simulink model "Bands6"  (R2018a)
settings: Solver=VariableStepAuto  StartTime=0.0  StopTime=0.01  RelTol=1e-3
undefined symbols (not defined in the file): fdesignblkfcn, G1, G2, G3, G4, G5, G6, gcbh, get, T
libraries: dspsrcs4 x1, dspxfrm3 x1, dspobslib x1
(part 2 of 2)

== system Bands6/Filter Bank /Filter 5/Bandpass Filter ==
  In : Inport
  Generated Filter Block : DiscreteFir  Tag=BlockMethodSubSystem  Coefficients=[5.80169645545239008e-08 -7.36943237726898499e-08 -1.75427224261787647e-07 6.43003652238008357e-07 -5.28400861014822699e-07 -1.09677006372124872e-06 3.31781145815797723e-06 -2.53629827715104648e-06 -3.9844890702122352e-06 1.18719656898654724e-05 -9.36329870334377579e-06 -1.03790001202894647e-05 3.33782074792234292e-05 -2.82688496798137121e-05 -2.05521184487442067e-05 7.80506937687390717e-05 -7.24051531518292809e-05 -3.00972665896463103e-05 0.000156331642592978074 -0.000161139708449589659 -2.51459625490565774e-05 0.00027208320875304079 -0.000316608173078618781 2.16589686587504518e-05 0.000412616192629136256 -0.000554862993402606202 0.000150692654732448582 0.000539329012231355752 -0.000872369046581383074 0.00040648652621871461 0.000585591917311480354 -0.00123249299141194816 0.000819163333665229158 0.000468918632894233629 -0.00156026749336166831 0.00138023742307578651 0.000120378783589651138 -0.00175423169147518113 0.0020230393593841569 -0.000474494460511202902 -0.00171910430407683527 0.00262123067921987652 -0.00123929489922535211 -0.00141248066958475638 0.00301527620477055891 -0.00199678966571106148 -0.000886619376992856694 0.00306523259567484602 -0.00250307330187033404 -0.000299861672526029936 0.00271252560159371226 -0.0025267776534030565 0.00012171384745463444 0.00202172673597837823 -0.00195008342165233677 0.000171258457679733067 0.00117467533990653263 -0.000848223237854478789 -0.000232692021354291518 0.000407587462984154323 0.00049828682517694795 -0.000971874699162834465 -8.85610034070924331e-05 0.00168202383752096766 -0.00173587675048004716 -0.000257954610305697056 0.00231927882960823771 -0.0021311939810607387 -0.000208481271414066242 0.00221255995829579624 -0.00186005918159203617 -0.000152015535511321729 0.00144662698791519725 -0.000889902743837175589 -0.000276867996253072691 0.000361608279357888897 0.000479878382522087887 -0.000618501588275072352 -0.000596003608316242437 0.00171105795524934576 -0.00100922150237675286 -0.00107795666262090685 0.00225971295712451125 -0.00115432392189464793 -0.000990924709133747398 0.00184772697412779606 -0.000811329556474037271 -0.000519796048615203871 0.000632035063372947707 2.24795851541013272e-05 -1.99606835156976085e-06 -0.000834109638794323189 0.00103494686315405552 0.000276818419330519436 -0.00185226591461002538 0.0017108115780006762 0.000244592720617982785 -0.00192809879322400628 0.00160075014399831887 6.14690263060736021e-05 -0.00103627337936797875 0.000611243434872120656 -1.91465685851059381e-05 0.000352130594981162352 -0.00086254312190905296 0.000142472563550124576 0.00151075077237486713 -0.00207507689699802569 0.000441166590936414166 0.00184666137896536179 -0.00230619796031119239 0.000576883090156487025 0.0012222015245354689 -0.00128685755170820796 0.000274230407592072759 2.27936196504474287e-05 0.000575424432464703099 -0.000466214697355777784 -0.0010743474392980398 0.00233874424726945645 -0.00127094741825165588 -0.00149764925353861132 0.00300421201905462943 -0.00156043086177853007 -0.00110627437447876828 0.00208716316600946047 -0.000919833301459701278 -0.000243179188607324851 -4.7857526112472211e-05 0.000546643345120831196 0.00051568179032762348 -0.00231508901657014434 0.00213514192708850938 0.000751567312124432063 -0.0034701576132279803 0.00285729371205205957 0.000471220012500609764 -0.00281293450406624882 0.00202632646388123307 6.63362851220782198e-05 -0.000623898569242482153 -0.000221229277446687944 -1.44191510628433379e-05 0.00194568773553285574 -0.00282840865428083277 0.00034940405710216229 0.00349933860496167174 -0.00429430022970904175 0.000800524320988185841 0.00319057761487220827 -0.00352540131711092655 0.000738596481679123563 0.00121803959086664378 -0.000585118425519459435 -0.000185229365218113291 -0.0012888920303765674 0.00315005677366268387 -0.00165923705179339448 -0.00294013727937736304 0.00562004228208647615 -0.00273360598608378934 -0.00290891244731987606 0.00522195115943085032 -0.00236421374140658282 -0.00139899652620957245 0.00182892903336386633 ...(+7522 chars)]  InputProcessing=Columns as channels (frame based)
  Out : Outport
  wires:
  In/1 -> Generated Filter Block/1
  Generated Filter Block/1 -> Out/1

== system Bands6/Filter Bank /Filter 6/Bandpass Filter ==
  In : Inport
  Generated Filter Block : DiscreteFir  Tag=BlockMethodSubSystem  Coefficients=[-8.46163060201177932e-08 4.43935124807243188e-07 -1.41960685880143677e-06 3.41720796909821398e-06 -6.66356512995420131e-06 1.08407356256788048e-05 -1.47502152166903733e-05 1.62989488752967176e-05 -1.30606215944798934e-05 3.47793268459825403e-06 1.16523753158832859e-05 -2.8158246186184923e-05 3.88640762038403156e-05 -3.59073795891534178e-05 1.46745586998780423e-05 2.21494551041817479e-05 -6.26963714884166994e-05 8.82752874711505939e-05 -8.04749647169068934e-05 3.10014021065765821e-05 5.01508359255908656e-05 -0.000133325946508563016 0.000177869540798289167 -0.000149597937610631751 4.05769804763433638e-05 0.000118706402074483244 -0.000263643793305792513 0.000318902583301029741 -0.000233976101207557848 1.54785793754956013e-05 0.000261673317368628204 -0.000475446213967466928 0.000507183945928171539 -0.000302117535111148827 -8.9147778119413865e-05 0.000513780824357670698 -0.000772340819809743035 0.00070904989012480742 -0.000297360294473450167 -0.000323673059816665851 0.000889607105286156145 -0.00112031835339431742 0.00085533138476342216 -0.000150635139510927289 -0.000717538205679782003 0.00135740149880777552 -0.00143743203462967997 0.000854983806421841328 0.00018714488152558458 -0.00124511234139790998 0.00182327158032334082 -0.00160782340572406955 0.000634007303107058675 0.000701600741107019643 -0.00180294955888707473 0.00214489216616386633 -0.0015275773663947841 0.000189556316408726272 0.00128379490726074829 -0.0022224637377778883 0.00218472951894835765 -0.00117084227052003352 -0.00036903116861821745 0.00174095357924741365 -0.00233077004155522391 0.00188942287316380708 -0.000642316941172821733 -0.000828092524053142135 0.00186514741688531506 -0.00204454974852675241 0.00135524746056228163 -0.000173209956407520876 -0.000946285101899397066 0.00154272513231569919 -0.00144986795240664582 0.000828753749831921921 -3.65034627839353723e-05 -0.000580574333915377162 0.000849696843853750268 -0.00080819571248590702 0.000613750534021326221 -0.000403516300384207339 0.000201838481981946407 6.35528708069222888e-05 -0.000454696350089640476 0.000909454914531755525 -0.00121455555550228889 0.00110568409962982003 -0.000447718480566853671 -0.000617005960404331481 0.00166305818073036733 -0.00215519913514135384 0.00172878074106186906 -0.000427356274822628731 -0.00124907872525232134 0.00254042937594043967 -0.00278870717640594505 0.00178542826189131867 8.48538036447978939e-05 -0.00199696610104887996 0.00307121781204429444 -0.00280244633710835219 0.00131131162609618955 0.000714272652850757566 -0.00235822881406850312 0.00291968995968195331 -0.00223259229715175051 0.000704702134780925329 0.000927069841760184326 -0.00197868268814773351 0.00212928233698165366 -0.00150667924986373379 0.000532256701158066118 0.000354516633408845589 -0.000916702383870690043 0.00116458580007394101 -0.00122818437264372729 0.00117533351036562257 -0.000923125336973821577 0.000317537789825255497 0.000671770547496120841 -0.00179153763622651565 0.00252690311856382417 -0.0023427212695793188 0.00102920537979640466 0.0010600858671846469 -0.00306019329961421376 0.00396581915002864379 -0.0031565953327821316 0.000793108626447434017 0.0021615656473172604 -0.0043520834700122718 0.00469015558993292423 -0.00292491990011144003 -0.000188327321990112864 0.00323100589929099184 -0.00481200079672475418 0.00424997037949580245 -0.0018904318332766555 -0.00110328188235767088 0.00336173806900166112 -0.00398710901746637553 0.00293769338447707942 -0.000938053261906044919 -0.00099410066962953166 0.00210602901458387289 -0.00223143872185789603 0.00172109040917809504 -0.0010787101446486304 0.000575164548669366096 -0.000108110138070809539 -0.000607274727426041156 0.00166923799585407136 -0.00273219514061845761 0.00309141239571915838 -0.00211205906069221938 -0.000248206287207592021 0.00318379226918635546 -0.0052918430608058821 0.0052700327924813245 -0.00270242960605342891 -0.00153612498702672385 0.00555777476386579497 -0.00734998824383596271 0.00583513844890293839 -0.00152032673105089496 -0.00365710607271531058 ...(+7570 chars)]  InputProcessing=Columns as channels (frame based)
  Out : Outport
  wires:
  In/1 -> Generated Filter Block/1
  Generated Filter Block/1 -> Out/1
